simulink model "Example_8_9"  (R2014a)
settings: Solver=FixedStepDiscrete  SolverMode=SingleTasking  StartTime=0.0  StopTime=10  RelTol=1e-3
libraries: dspsrcs4 x1, dsparch4 x1
settings Model: Creator=Lee Edwards  LastModifiedBy=Lee
settings DataIOCC: SignalLoggingSaveFormat=ModelDataLogs  SaveOutput=off  SignalLogging=off  SaveTime=off
settings OptimizationCC: ExpressionDepthLimit=2147483647
settings DebuggingCC: AlgebraicLoopMsg=error  UnderspecifiedInitializationDetection=Classic  SingleTaskRateTransMsg=error  FcnCallInpInsideContextMsg=UseLocalSettings  StateNameClashWarn=warning
settings GRTTargetCC: CombineOutputUpdateFcns=off  GRTInterface=on

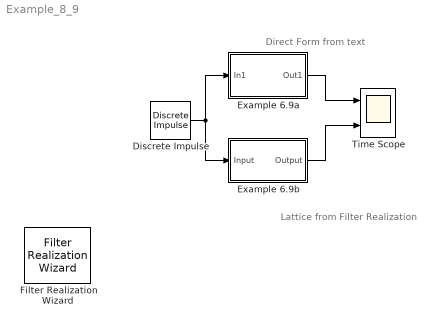
== system Example_8_9 ==
  note: Direct Form from text
  note: Lattice from Filter Realization
  Discrete Impulse : dspsrcs4/Discrete  Impulse  Delay=0  SampleTime=1  FrameSample=1  dataType=double  isSigned=on  wordLen=16  udDataType=sfix(16)  fracBitsMode=Best precision  numFracBits=15  OutDataTypeStr=double  LastOutDataTypeStr=double
  Example 6.9a : Subsystem
  Example 6.9b : Subsystem  Tag=FilterWizardSubSystem
      settings: ErrorFcn=dspFilterRealizedInBasicElemsAlgLoopErrFcnCallback
  Filter Realization Wizard : dsparch4/Filter Realization Wizard
  Time Scope : Scope  NumInputPorts=2
      settings: YMin=-2~-2  YMax=2~2  DataFormat=Structure
  wires:
  Discrete Impulse/1 -> Example 6.9a/1(In1), Example 6.9b/1(Input)
  Example 6.9a/1(Out1) -> Time Scope/1
  Example 6.9b/1(Output) -> Time Scope/2

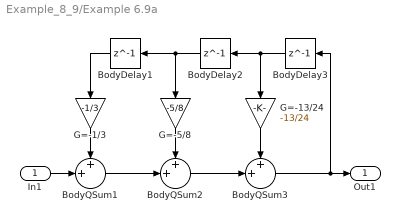
== system Example_8_9/Example 6.9a ==
  In1 : Inport
  BodyDelay1 : Delay  DelayLength=1  InputProcessing=Inherited
  BodyDelay2 : Delay  DelayLength=1  InputProcessing=Inherited
  BodyDelay3 : Delay  DelayLength=1  InputProcessing=Inherited
  BodyQSum1 : Sum  Inputs=++|  RndMeth=Nearest  SaturateOnIntegerOverflow=on  OutDataTypeStr=Inherit: Same as first input
  BodyQSum2 : Sum  Inputs=++|  RndMeth=Nearest  SaturateOnIntegerOverflow=on  OutDataTypeStr=Inherit: Same as first input
  BodyQSum3 : Sum  Inputs=++|  RndMeth=Nearest  SaturateOnIntegerOverflow=on  OutDataTypeStr=Inherit: Same as first input
  G=-1/3 : Gain  Gain=-1/3  ParamDataTypeStr=float('double')  RndMeth=Nearest  SaturateOnIntegerOverflow=on  OutDataTypeStr=Inherit: Same as input
  G=-13/24 : Gain  Gain=-13/24  ParamDataTypeStr=float('double')  RndMeth=Nearest  SaturateOnIntegerOverflow=on  OutDataTypeStr=Inherit: Same as input
  G=-5/8 : Gain  Gain=-5/8  ParamDataTypeStr=float('double')  RndMeth=Nearest  SaturateOnIntegerOverflow=on  OutDataTypeStr=Inherit: Same as input
  Out1 : Outport
  wires:
  BodyDelay2/1 -> BodyDelay1/1, G=-5/8/1
  BodyDelay3/1 -> BodyDelay2/1, G=-13/24/1
  BodyDelay1/1 -> G=-1/3/1
  G=-1/3/1 -> BodyQSum1/1
  G=-5/8/1 -> BodyQSum2/1
  G=-13/24/1 -> BodyQSum3/1
  BodyQSum1/1 -> BodyQSum2/2
  BodyQSum2/1 -> BodyQSum3/2
  BodyQSum3/1 -> BodyDelay3/1, Out1/1
  In1/1 -> BodyQSum1/2

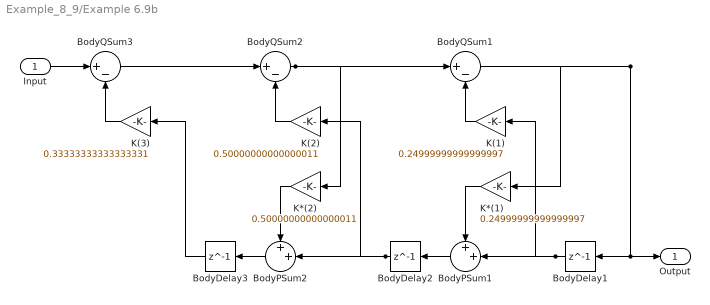
== system Example_8_9/Example 6.9b ==
  Input : Inport
  BodyDelay1 : Delay  DelayLength=1  InputProcessing=Inherited
  BodyDelay2 : Delay  DelayLength=1  InputProcessing=Inherited
  BodyDelay3 : Delay  DelayLength=1  InputProcessing=Inherited
  BodyPSum1 : Sum  Inputs=++|  RndMeth=Nearest  SaturateOnIntegerOverflow=on  OutDataTypeStr=Inherit: Same as first input
  BodyPSum2 : Sum  Inputs=++|  RndMeth=Nearest  SaturateOnIntegerOverflow=on  OutDataTypeStr=Inherit: Same as first input
  BodyQSum1 : Sum  Inputs=|+-  RndMeth=Nearest  SaturateOnIntegerOverflow=on  OutDataTypeStr=Inherit: Same as first input
  BodyQSum2 : Sum  Inputs=|+-  RndMeth=Nearest  SaturateOnIntegerOverflow=on  OutDataTypeStr=Inherit: Same as first input
  BodyQSum3 : Sum  Inputs=|+-  RndMeth=Nearest  SaturateOnIntegerOverflow=on  OutDataTypeStr=Inherit: Same as first input
  K(1) : Gain  Gain=0.24999999999999997  ParamDataTypeStr=float('double')  RndMeth=Nearest  SaturateOnIntegerOverflow=on  OutDataTypeStr=Inherit: Same as input
  K(2) : Gain  Gain=0.50000000000000011  ParamDataTypeStr=float('double')  RndMeth=Nearest  SaturateOnIntegerOverflow=on  OutDataTypeStr=Inherit: Same as input
  K(3) : Gain  Gain=0.33333333333333331  ParamDataTypeStr=float('double')  RndMeth=Nearest  SaturateOnIntegerOverflow=on  OutDataTypeStr=Inherit: Same as input
  K*(1) : Gain  Gain=0.24999999999999997  ParamDataTypeStr=float('double')  RndMeth=Nearest  SaturateOnIntegerOverflow=on  OutDataTypeStr=Inherit: Same as input
  K*(2) : Gain  Gain=0.50000000000000011  ParamDataTypeStr=float('double')  RndMeth=Nearest  SaturateOnIntegerOverflow=on  OutDataTypeStr=Inherit: Same as input
  Output : Outport
  wires:
  K(1)/1 -> BodyQSum1/2
  K*(1)/1 -> BodyPSum1/1
  BodyPSum1/1 -> BodyDelay2/1
  BodyDelay1/1 -> K(1)/1, BodyPSum1/2
  BodyQSum2/1 -> K*(2)/1, BodyQSum1/1
  K(2)/1 -> BodyQSum2/2
  K*(2)/1 -> BodyPSum2/1
  BodyPSum2/1 -> BodyDelay3/1
  BodyDelay2/1 -> K(2)/1, BodyPSum2/2
  BodyQSum3/1 -> BodyQSum2/1
  K(3)/1 -> BodyQSum3/2
  BodyDelay3/1 -> K(3)/1
  Input/1 -> BodyQSum3/1
  BodyQSum1/1 -> K*(1)/1, BodyDelay1/1, Output/1
